simulink model "SDsimRLC_closed"  (R2018b)
settings: Solver=ode4  StartTime=0.0  StopTime=11e-3*0+0.05*2*1  FixedStep=Tsim  MaxStep=1e-4  RelTol=1e-6
values from neighbouring files (symbols this model uses):
  C = 100e-6    (= 0.0001)    [closedRLC_init.m]
  fsw = PWM_frequency    (= 10000)    [closedRLC_init.m]
  imax = 2    [closedRLC_init.m]
  ki = 33.35    [closedRLC_init.m]
  kp = 0.0047    [closedRLC_init.m]
  L = 860e-6    (= 0.00086)    [closedRLC_init.m]
  Rc = 66e-3    (= 0.066)    [closedRLC_init.m]
  Rl = 0.15    [closedRLC_init.m]
  Ro = 6.8    [closedRLC_init.m]
  Ts = Tsw    (= 0.0001)    [closedRLC_init.m]
  Tsim = Tsw/400    (= 2.5e-07)    [closedRLC_init.m]
  Vdc = 15    [closedRLC_init.m]
libraries: powerlib x19, simulink x5
settings Model: Creator=mattia  LastModifiedBy=matti
settings DataIOCC: ReturnWorkspaceOutputs=on

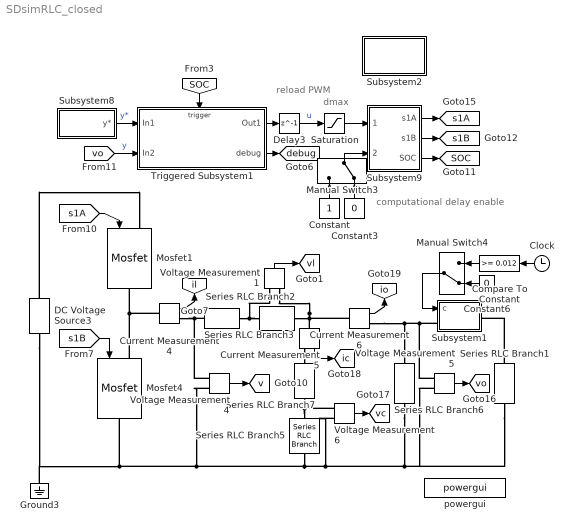
== system SDsimRLC_closed ==
  note: reload
      | PWM
  note: dmax
  note: computational delay
      | enable
  Clock : Clock
  Compare To Constant : simulink/Logic and Bit Operations/Compare To Constant  relop=>=  const=0.012  OutDataTypeStr=boolean
  Constant : Constant  SampleTime=Ts
  Constant3 : Constant  Value=0  SampleTime=Ts
  Constant6 : Constant  Value=0  SampleTime=Ts
  Current Measurement4 : powerlib/Measurements/Current Measurement  PhasorSimulation=off  OutputType=Complex  PSBequivalent=0
  Current Measurement5 : powerlib/Measurements/Current Measurement  PhasorSimulation=off  OutputType=Complex  PSBequivalent=0
  Current Measurement6 : powerlib/Measurements/Current Measurement  PhasorSimulation=off  OutputType=Complex  PSBequivalent=0
  DC Voltage Source3 : powerlib/Electrical Sources/DC Voltage Source  Amplitude=Vdc  Measurements=None
      settings: SourceProductName=Simscape Electrical
  Delay3 : Delay  DelayLength=1  SampleTime=Ts/2
  Ground3 : powerlib/Elements/Ground  LConnTagsString=a
      settings: SourceProductName=Simscape Electrical
  Manual Switch3 : ManualSwitch  CurrentSetting=0
  Manual Switch4 : ManualSwitch  CurrentSetting=0
  Mosfet1 : powerlib/Power Electronics/Mosfet  Ron=0.1  Lon=0  Rd=0.01  Vfd=0  IC=0  Rs=1e5  Cs=inf  Measurements=off
      settings: SourceProductName=Simscape Electrical
  Mosfet4 : powerlib/Power Electronics/Mosfet  Ron=0.1  Lon=0  Rd=0.01  Vfd=0  IC=0  Rs=1e5  Cs=inf  Measurements=off
      settings: SourceProductName=Simscape Electrical
  Saturation : Saturate  UpperLimit=1  LowerLimit=0
  Series RLC Branch1 : powerlib/Elements/Series RLC Branch  LConnTagsString=__new0  RConnTagsString=__new0  BranchType=R  Resistance=Ro  Inductance=L  SetiL0=off  InitialCurrent=0.1  Capacitance=1e-6  Setx0=off  InitialVoltage=0  Measurements=None
  Series RLC Branch2 : powerlib/Elements/Series RLC Branch  LConnTagsString=__new0  RConnTagsString=__new0  BranchType=L  Resistance=Rl  Inductance=L  SetiL0=off  InitialCurrent=0.1  Capacitance=1e-6  Setx0=off  InitialVoltage=0  Measurements=None
  Series RLC Branch3 : powerlib/Elements/Series RLC Branch  LConnTagsString=__new0  RConnTagsString=__new0  BranchType=R  Resistance=Rl  Inductance=L  SetiL0=off  InitialCurrent=0.1  Capacitance=1e-6  Setx0=off  InitialVoltage=0  Measurements=None
  Series RLC Branch5 : powerlib/Elements/Series RLC Branch  LConnTagsString=__new0  RConnTagsString=__new0  BranchType=C  Resistance=Ro+Rl  Inductance=L  SetiL0=off  InitialCurrent=0.1  Capacitance=C  Setx0=off  InitialVoltage=0  Measurements=None
  Series RLC Branch6 : powerlib/Elements/Series RLC Branch  LConnTagsString=__new0  RConnTagsString=__new0  BranchType=R  Resistance=Ro  Inductance=L  SetiL0=off  InitialCurrent=0.1  Capacitance=1e-6  Setx0=off  InitialVoltage=0  Measurements=None
  Series RLC Branch7 : powerlib/Elements/Series RLC Branch  LConnTagsString=__new0  RConnTagsString=__new0  BranchType=R  Resistance=Rc  Inductance=L  SetiL0=off  InitialCurrent=0.1  Capacitance=1e-6  Setx0=off  InitialVoltage=0  Measurements=None
  Subsystem1 : Subsystem
      mask Display: disp('circuit\nbreaker')
  Subsystem2 : Subsystem
      mask Display: disp('stream')
  Subsystem8 : Subsystem
      mask Display: disp('reference')
  Subsystem9 : Subsystem
      mask Display: disp('modulator')
  Triggered Subsystem1 : Subsystem  TreatAsAtomicUnit=on
      mask Display: disp('current controller\n(syncronized with PWM)')
  Voltage Measurement{1,4..6} (4 alike) : powerlib/Measurements/Voltage Measurement  PhasorSimulation=off  OutputType=Complex  PSBequivalent=0
  powergui : powerlib/powergui  Priority=1  SimulationMode=Continuous  SampleTime=Tsim  frequency=60  Iterations=50  frequencyindice=0  Pbase=100e6  ErrMax=1e-4  UnitsV=kV  UnitsW=MW  buscounter=0  FunctionMessages=on  echomessages=off  EnableUseOfTLC=off  CurrentSourceSwitches=off  DisableSnubberDevices=on  DisableRonSwitches=on  DisableVfSwitches=on  DisplayEquations=off  SolverType=Tustin/Backward Euler (TBE)  Interpol=off  ExternalGateDelay=off  methode=off  Ts=100  x0status=blocks  SPID=off  SwTol=0  HookPort=off  RestoreLinks=warning  ResistiveCurrentMeasurement=off  Frange=[0:2:500]  Ylog=off  Xlog=on  ShowGrid=off  save=off  variable=ZData  structure=0  ZoomFFT=off  StartTime=0.0  cycles=1  DisplayStyle=1  fundamental=60  FreqAxis=off  MaxFrequency=1000  frequencyindicesteady=1  RmsSteady=1  display=off
  tag scope: SOC=global, debug=global, ic=global, il=global, io=global, s1A=global, s1B=global, v=global, vc=global, vl=global, vo=global
  wires:
  Triggered Subsystem1/1(Out1) -> Delay3/1
  Constant3/1 -> Manual Switch3/2
  Manual Switch3/1 -> Subsystem9/2(enable delay)
  [vo] -> Triggered Subsystem1/2(In2)  "y"
  Triggered Subsystem1/2(debug) -> [debug]
  Subsystem9/1(s1A) -> [s1A]
  Subsystem9/2(s1B) -> [s1B]
  Voltage Measurement4/1 -> [v]
  [s1B] -> Mosfet4/1
  Saturation/1 -> Subsystem9/1(modA)
  Subsystem9/3(SOC) -> [SOC]
  [s1A] -> Mosfet1/1
  Subsystem8/1(y*) -> Triggered Subsystem1/1(In1)  "y*"
  Constant/1 -> Manual Switch3/1
  Delay3/1 -> Saturation/1  "u"
  Current Measurement4/1 -> [il]
  [SOC] -> Triggered Subsystem1/Trigger
  Voltage Measurement5/1 -> [vo]
  Compare To Constant/1 -> Manual Switch4/1
  Constant6/1 -> Manual Switch4/2
  Voltage Measurement6/1 -> [vc]
  Current Measurement5/1 -> [ic]
  Current Measurement6/1 -> [io]
  Manual Switch4/1 -> Subsystem1/1(c)
  Clock/1 -> Compare To Constant/1
  Voltage Measurement1/1 -> [vl]
  connections:
  Mosfet4/LConn1 -- Mosfet1/RConn1 -- Current Measurement4/LConn1
  Voltage Measurement4/LConn1 -- Series RLC Branch3/LConn1 -- Current Measurement4/RConn1
  Voltage Measurement4/LConn2 -- Series RLC Branch1/RConn1 -- Voltage Measurement5/LConn2 -- Series RLC Branch6/RConn1 -- Voltage Measurement6/LConn2 -- Series RLC Branch5/RConn1 -- DC Voltage Source3/LConn1 -- Ground3/LConn1 -- Mosfet4/RConn1
  DC Voltage Source3/RConn1 -- Mosfet1/LConn1
  Current Measurement5/LConn1 -- Series RLC Branch2/RConn1 -- Current Measurement6/LConn1 -- Voltage Measurement1/LConn2
  Series RLC Branch1/LConn1 -- Subsystem1/RConn1
  Series RLC Branch7/RConn1 -- Series RLC Branch5/LConn1 -- Voltage Measurement6/LConn1
  Current Measurement5/RConn1 -- Series RLC Branch7/LConn1
  Voltage Measurement5/LConn1 -- Subsystem1/LConn1 -- Current Measurement6/RConn1 -- Series RLC Branch6/LConn1
  Series RLC Branch3/RConn1 -- Voltage Measurement1/LConn1 -- Series RLC Branch2/LConn1

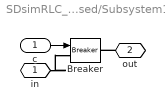
== system SDsimRLC_closed/Subsystem1 ==
  c : Inport
  Breaker : powerlib/Elements/Breaker  InitialState=0  SwitchingTimes="[1/60  5/60]"  External=on  BreakerResistance=1e-4  SnubberResistance=1e6  SnubberCapacitance=inf  Measurements=None  MoreParameters=on  NoBreakLoop=off
      settings: SourceProductName=Simscape Power Systems
  in : PMIOPort  Side=Left
  out : PMIOPort  Port=2  Side=Right
  wires:
  c/1 -> Breaker/1
  connections:
  in/RConn1 -- Breaker/LConn1
  out/RConn1 -- Breaker/RConn1

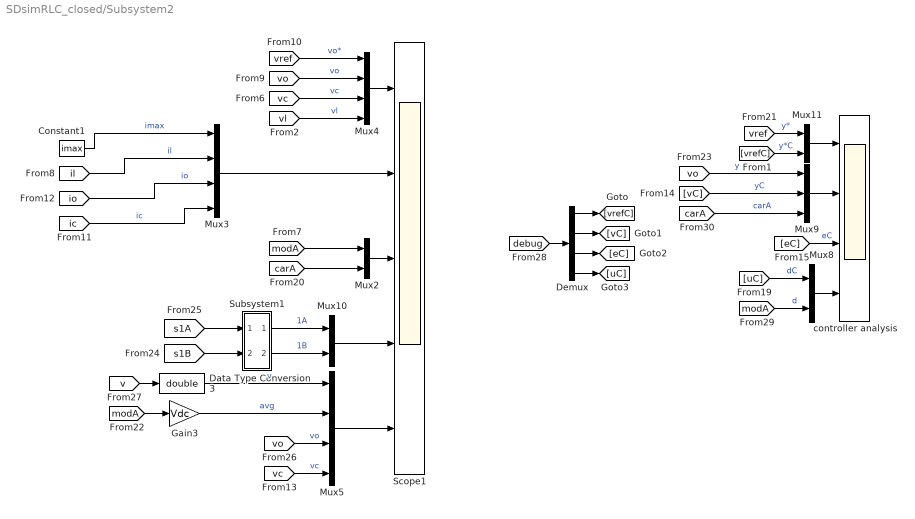
== system SDsimRLC_closed/Subsystem2 ==
  Constant1 : Constant  Value=imax
  Data Type Conversion3 : DataTypeConversion  OutDataTypeStr=double
  Demux : Demux
  Gain3 : Gain  Gain=Vdc
  Mux{2,8,10..11} (4 alike) : Mux  Inputs=2
  Mux3 : Mux
  Mux4 : Mux
  Mux5 : Mux
  Mux9 : Mux  Inputs=3
  Scope1 : Scope  NumInputPorts=5
  Subsystem1 : Subsystem
      mask Display: disp('shift')
  controller analysis : Scope  NumInputPorts=4
  wires:
  Mux4/1 -> Scope1/1
  [vo] -> Mux4/2  "vo"
  [vref] -> Mux4/1  "vo*"
  Constant1/1 -> Mux3/1  "imax"
  [il] -> Mux3/2  "il"
  Mux3/1 -> Scope1/2
  [ic] -> Mux3/4  "ic"
  [io] -> Mux3/3  "io"
  [vc] -> Mux5/4  "vc"
  [vc] -> Mux4/3  "vc"
  [modA] -> Mux2/1
  [carA] -> Mux2/2
  Mux2/1 -> Scope1/3
  [vo] -> Mux5/3  "vo"
  [s1A] -> Subsystem1/1(In1)
  Subsystem1/2(Out2) -> Mux10/2  "1B"
  Mux10/1 -> Scope1/4
  Subsystem1/1(Out1) -> Mux10/1  "1A"
  Gain3/1 -> Mux5/2  "avg"
  [s1B] -> Subsystem1/2(In2)
  [v] -> Data Type Conversion3/1
  Mux5/1 -> Scope1/5
  [modA] -> Gain3/1
  Data Type Conversion3/1 -> Mux5/1  "v"
  [carA] -> Mux9/3  "carA"
  Mux9/1 -> controller analysis/2
  [debug] -> Demux/1
  Demux/2 -> [vC]
  Demux/4 -> [uC]
  Demux/3 -> [eC]
  [modA] -> Mux8/2  "d"
  [vrefC] -> Mux11/2  "y*C"
  [uC] -> Mux8/1  "dC"
  [vref] -> Mux11/1  "y*"
  Demux/1 -> [vrefC]
  [vC] -> Mux9/2  "yC"
  [vo] -> Mux9/1  "y"
  [eC] -> controller analysis/3  "eC"
  Mux8/1 -> controller analysis/4
  Mux11/1 -> controller analysis/1
  [vl] -> Mux4/4  "vl"

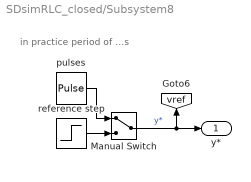
== system SDsimRLC_closed/Subsystem8 ==
  note: in practice period of ...s
  Manual Switch : ManualSwitch
  pulses : DiscretePulseGenerator  Amplitude=6  Period=500  PulseWidth=250  PhaseDelay=5  SampleTime=Ts
  reference step : Step  Time=5*Ts  After=6  SampleTime=Ts
  y* : Outport
  tag scope: vref=global
  wires:
  Manual Switch/1 -> [vref], y*/1  "y*"
  reference step/1 -> Manual Switch/2
  pulses/1 -> Manual Switch/1

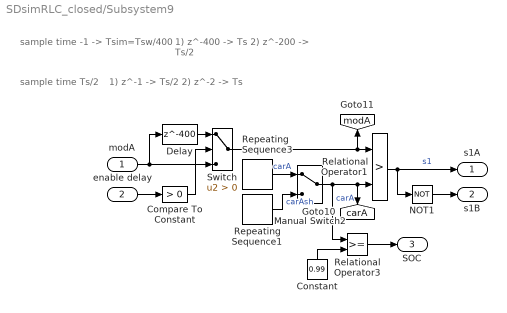
== system SDsimRLC_closed/Subsystem9 ==
  note: sample time Ts/2
  note: 1)  z^-1 -> Ts/2
      | 2)  z^-2 -> Ts
  note: sample time -1 -> Tsim=Tsw/400
  note: 1)  z^-400 -> Ts
      | 2)  z^-200 -> Ts/2
  modA : Inport
  enable delay : Inport  Port=2
  Compare To Constant : simulink/Logic and Bit Operations/Compare To Constant  relop=>  const=0  OutDataTypeStr=boolean
  Constant : Constant  Value=0.99  SampleTime=Ts
  Delay : Delay  DelayLength=400  SampleTime=Tsim
  Manual Switch2 : ManualSwitch
  NOT1 : Logic  Operator=NOT  IconShape=distinctive  AllPortsSameDT=off  OutDataTypeStr=boolean
  Relational Operator1 : RelationalOperator  Operator=>  OutDataTypeStr=boolean  RndMeth=Simplest
  Relational Operator3 : RelationalOperator  OutDataTypeStr=boolean  RndMeth=Simplest
  Repeating Sequence1 : simulink/Sources/Repeating Sequence  rep_seq_t=[0 1/(4*fsw) 1/(2*fsw) 3/(4*fsw) 1/fsw]  rep_seq_y=[0.5 0 0.5 1 0.5]
  Repeating Sequence3 : simulink/Sources/Repeating Sequence  rep_seq_t=[0 1/(2*fsw) 1/fsw]  rep_seq_y=[0 1 0]
  Switch : Switch  Criteria=u2 > Threshold
  s1A : Outport
  s1B : Outport  Port=2
  SOC : Outport  Port=3
  tag scope: carA=global, modA=global
  wires:
  Manual Switch2/1 -> Relational Operator3/1, [carA], Relational Operator1/2  "carA"
  Relational Operator1/1 -> NOT1/1, s1A/1  "s1"
  Repeating Sequence1/1 -> Manual Switch2/2  "carAsh"
  Repeating Sequence3/1 -> Manual Switch2/1  "carA"
  NOT1/1 -> s1B/1
  Constant/1 -> Relational Operator3/2
  Delay/1 -> Switch/1
  Compare To Constant/1 -> Switch/2
  modA/1 -> Delay/1, Switch/3
  enable delay/1 -> Compare To Constant/1
  Relational Operator3/1 -> SOC/1
  Switch/1 -> [modA], Relational Operator1/1

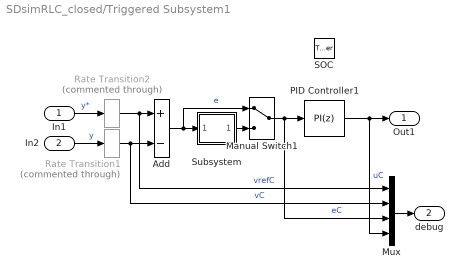
== system SDsimRLC_closed/Triggered Subsystem1 ==
  In1 : Inport
  In2 : Inport  Port=2
  SOC : TriggerPort  VariantControl=Variant
  Add : Sum  Inputs=+-
  Manual Switch1 : ManualSwitch
  Mux : Mux
  PID Controller1 : simulink/Continuous/PID Controller  Controller=PI  Form=Parallel  TimeDomain=Discrete-time  SampleTime=-1  IntegratorMethod=Backward Euler  FilterMethod=Forward Euler  ControllerParametersSource=internal  P=kp  I=ki  D=0  UseFilter=on  N=100  TunerSelectOption=Transfer Function Based (PID Tuner App)  ZeroCross=off  InitialConditionSource=internal  InitialConditionForIntegrator=0  InitialConditionForFilter=0  DifferentiatorICPrevScaledInput=0  ExternalReset=none  TrackingMode=off  Kt=1  LimitOutput=on  UpperSaturationLimit=0.98  LowerSaturationLimit=0  LinearizeAsGain=on  AntiWindupMode=back-calculation  Kb=ki/kp  POutMin=[]  POutMax=[]  IOutMin=[]  IOutMax=[]  DOutMin=[]  DOutMax=[]  NOutMin=[]  NOutMax=[]  SumOutMin=[]  SumOutMax=[]  SaturationOutMin=[]  SaturationOutMax=[]  PParamMin=[]  PParamMax=[]  IParamMin=[]  IParamMax=[]  DParamMin=[]  DParamMax=[]  NParamMin=[]  NParamMax=[]  KbParamMin=[]  KbParamMax=[]  KtParamMin=[]  KtParamMax=[]  KbOutMin=[]  KbOutMax=[]  KtOutMin=[]  KtOutMax=[]  IntegratorOutMin=[]  IntegratorOutMax=[]  FilterOutMin=[]  FilterOutMax=[]  SumI1OutMin=[]  SumI1OutMax=[]  SumI2OutMin=[]  SumI2OutMax=[]  SumI3OutMin=[]  SumI3OutMax=[]  SumI4OutMin=[]  SumI4OutMax=[]  SumDOutMin=[]  SumDOutMax=[]  DifferentiatorOutMin=[]  DifferentiatorOutMax=[]  FilterDiffOutCoefMin=[]  FilterDiffOutCoefMax=[]  ReciprocalOutMin=[]  ReciprocalOutMax=[]  SumDenOutMin=[]  SumDenOutMax=[]  SumNumOutMin=[]  SumNumOutMax=[]  DivideOutMin=[]  DivideOutMax=[]  IntegratorContinuousStateAttributes=''  IntegratorStateMustResolveToSignalObject=off  IntegratorRTWStateStorageClass=Auto  FilterContinuousStateAttributes=''  FilterStateMustResolveToSignalObject=off  FilterRTWStateStorageClass=Auto  ParallelPVariant=InternalParameters  IdealPVariant=Disabled  IVariant=InternalParameters  DVariant=Disabled  IntegratorVariant=Discrete  SatVariant=Enabled  AWVariant=BackCalculation  PCopyVariant=Disabled  TRVariant=Disabled  FdbkBlocksVariant=Feedback  IdealPFdbkVariant=Passthrough  SatFdbkVariant=Enabled  DerivativeFilterVariant=Disabled  NVariant=Disabled  NCopyVariant=Disabled_SignalSpec  FilterICVariant=Disabled  IntegratorICVariant=InternalICs  ExternalResetVariant=Disabled  TRSumVariant=Passthrough  SumFdbkVariant=Enabled  SumVariant=Sum_PI
  Rate Transition1 : RateTransition  Commented=through  OutPortSampleTime=Ts
  Rate Transition2 : RateTransition  Commented=through  OutPortSampleTime=Ts
  Subsystem : Subsystem
      mask Display: disp('cut\nnoise')
  Out1 : Outport
  debug : Outport  Port=2
  wires:
  In2/1 -> Rate Transition1/1  "y"
  Manual Switch1/1 -> Mux/3, PID Controller1/1  "eC"
  Rate Transition2/1 -> Mux/1, Add/1  "vrefC"
  In1/1 -> Rate Transition2/1  "y*"
  PID Controller1/1 -> Out1/1, Mux/4  "uC"
  Rate Transition1/1 -> Add/2, Mux/2  "vC"
  Mux/1 -> debug/1
  Add/1 -> Manual Switch1/1, Subsystem/1(In1)  "e"
  Subsystem/1(Out1) -> Manual Switch1/2

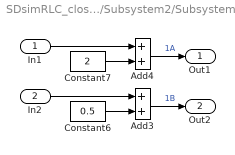
== system SDsimRLC_closed/Subsystem2/Subsystem1 ==
  In1 : Inport
  In2 : Inport  Port=2
  Add3 : Sum
  Add4 : Sum
  Constant6 : Constant  Value=0.5  VectorParams1D=off  SampleTime=-1
  Constant7 : Constant  Value=2  SampleTime=-1
  Out1 : Outport
  Out2 : Outport  Port=2
  wires:
  Add3/1 -> Out2/1  "1B"
  Add4/1 -> Out1/1  "1A"
  Constant7/1 -> Add4/2
  Constant6/1 -> Add3/2
  In1/1 -> Add4/1
  In2/1 -> Add3/1

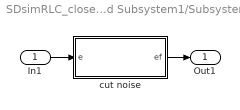
== system SDsimRLC_closed/Triggered Subsystem1/Subsystem ==
  In1 : Inport
  cut noise : MATLAB Function  TreatAsAtomicUnit=on
  Out1 : Outport
  wires:
  In1/1 -> cut noise/1(e)
  cut noise/1(ef) -> Out1/1

== matlab function SDsimRLC_closed/Triggered Subsystem1/Subsystem/cut noise ==
  data: e input; ef output
function ef = cutter(e)
if e <= 0.03 && e >= 0
    ef = 0;
elseif e >= -0.03 && e < 0
    ef = 0;
else
    ef = e;
end
